simulink model "High_level_control_system"  (R2022b)
settings: Solver=VariableStepAuto  StartTime=0.0  StopTime=10.0  RelTol=1e-3
settings Model: Creator=louis  LastModifiedBy=simon
settings DebuggingCC: UnconnectedInputMsg=warning  UnconnectedOutputMsg=warning  UnconnectedLineMsg=warning
settings ModelReferenceCC: EnableRefExpFcnMdlSchedulingChecks=on
settings RTWCC: DLArmComputeVersion=19.05

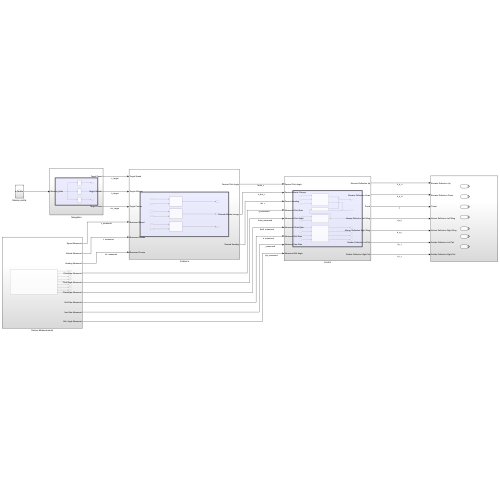
[thumbnail: Simulink's stored preview of the top-level diagram]
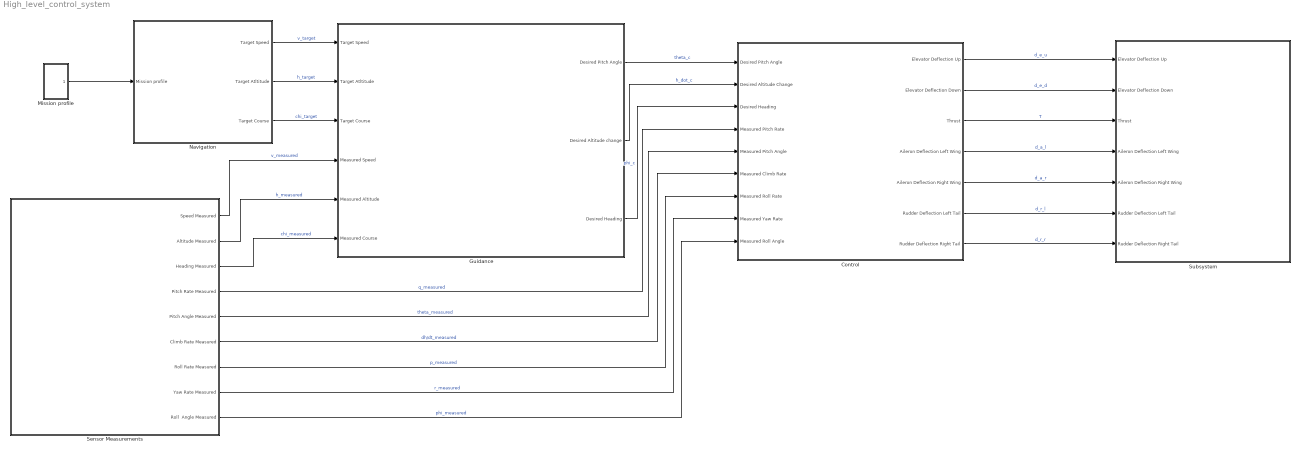
== system High_level_control_system ==
  Control : Subsystem
  Guidance : Subsystem
  Mission profile : Subsystem
  Navigation : Subsystem
  Sensor Measurements : Subsystem
  Subsystem : Subsystem
  wires:
  Navigation/1(Target Speed) -> Guidance/1(Target Speed)  "v_target"
  Navigation/2(Target Atltitude) -> Guidance/2(Target Atltitude)  "h_target"
  Navigation/3(Target Course) -> Guidance/3(Target Course)  "chi_target"
  Guidance/3(Desired Heading) -> Control/3(Desired Heading)  "phi_c"
  Guidance/2(Desired Altitude change) -> Control/2(Desired Altitude Change)  "h_dot_c"
  Guidance/1(Desired Pitch Angle) -> Control/1(Desired Pitch Angle)  "theta_c"
  Control/1(Elevator Deflection Up) -> Subsystem/1(Elevator Deflection Up)  "d_e_u"
  Control/3(Thrust) -> Subsystem/3(Thrust)  "T"
  Control/2(Elevator Deflection Down) -> Subsystem/2(Elevator Deflection Down)  "d_e_d"
  Control/4(Aileron Deflection Left Wing) -> Subsystem/4(Aileron Deflection Left Wing)  "d_a_l"
  Control/6(Rudder Deflection Left Tail) -> Subsystem/6(Rudder Deflection Left Tail)  "d_r_l"
  Control/5(Aileron Deflection Right Wing) -> Subsystem/5(Aileron Deflection Right Wing)  "d_a_r"
  Control/7(Rudder Deflection Right Tail) -> Subsystem/7(Rudder Deflection Right Tail)  "d_r_r"
  Sensor Measurements/1(Speed Measured) -> Guidance/4(Measured Speed)  "v_measured"
  Sensor Measurements/5(Pitch Angle Measured) -> Control/5(Measured Pitch Angle)  "theta_measured"
  Sensor Measurements/4(Pitch Rate Measured) -> Control/4(Measured Pitch Rate)  "q_measured"
  Sensor Measurements/3(Heading Measured) -> Guidance/6(Measured Course)  "chi_measured"
  Sensor Measurements/7(Roll Rate Measured) -> Control/7(Measured Roll Rate)  "p_measured"
  Sensor Measurements/8(Yaw Rate Measured) -> Control/8(Measured Yaw Rate)  "r_measured"
  Sensor Measurements/2(Altitude Measured) -> Guidance/5(Measured Altitude)  "h_measured"
  Sensor Measurements/9(Roll  Angle Measured) -> Control/9(Measured Roll Angle)  "phi_measured"
  Sensor Measurements/6(Climb Rate Measured) -> Control/6(Measured Climb Rate)  "dh/dt_measured"
  Mission profile/1(Mission profile) -> Navigation/1(Mission profile)

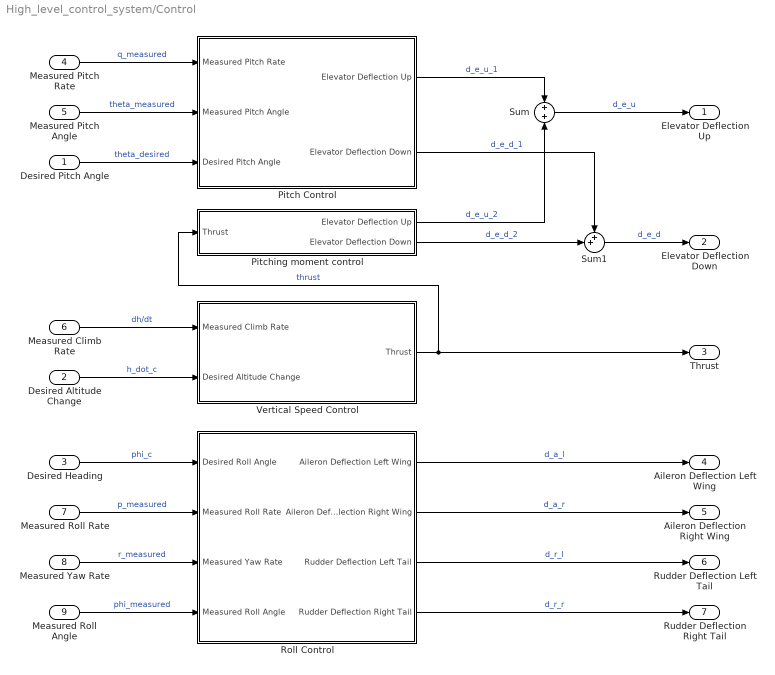
== system High_level_control_system/Control ==
  Desired Pitch Angle : Inport
  Desired Altitude Change : Inport  Port=2
  Desired Heading : Inport  Port=3
  Measured Pitch Rate : Inport  Port=4
  Measured Pitch Angle : Inport  Port=5
  Measured Climb Rate : Inport  Port=6
  Measured Roll Rate : Inport  Port=7
  Measured Yaw Rate : Inport  Port=8
  Measured Roll Angle : Inport  Port=9
  Pitch Control : Subsystem
  Pitching moment control : Subsystem
  Roll Control : Subsystem
  Sum : Sum
  Sum1 : Sum  Inputs=++|
  Vertical Speed Control : Subsystem
  Elevator Deflection Up : Outport
  Elevator Deflection Down : Outport  Port=2
  Thrust : Outport  Port=3
  Aileron Deflection Left Wing : Outport  Port=4
  Aileron Deflection Right Wing : Outport  Port=5
  Rudder Deflection Left Tail : Outport  Port=6
  Rudder Deflection Right Tail : Outport  Port=7
  wires:
  Pitch Control/1(Elevator Deflection Up) -> Sum/1  "d_e_u_1"
  Measured Pitch Rate/1 -> Pitch Control/1(Measured Pitch Rate)  "q_measured"
  Measured Pitch Angle/1 -> Pitch Control/2(Measured Pitch Angle)  "theta_measured"
  Desired Pitch Angle/1 -> Pitch Control/3(Desired Pitch Angle)  "theta_desired"
  Vertical Speed Control/1(Thrust) -> Pitching moment control/1(Thrust), Thrust/1  "thrust"
  Pitching moment control/1(Elevator Deflection Up) -> Sum/2  "d_e_u_2"
  Measured Climb Rate/1 -> Vertical Speed Control/1(Measured Climb Rate)  "dh/dt"
  Desired Altitude Change/1 -> Vertical Speed Control/2(Desired Altitude Change)  "h_dot_c"
  Desired Heading/1 -> Roll Control/1("Desired Roll Angle ")  "phi_c"
  Measured Roll Rate/1 -> Roll Control/2(Measured Roll Rate)  "p_measured"
  Measured Yaw Rate/1 -> Roll Control/3(Measured Yaw Rate)  "r_measured"
  Measured Roll Angle/1 -> Roll Control/4(Measured Roll Angle)  "phi_measured"
  Roll Control/3(Rudder Deflection Left Tail) -> Rudder Deflection Left Tail/1  "d_r_l"
  Roll Control/1(Aileron Deflection Left Wing) -> Aileron Deflection Left Wing/1  "d_a_l"
  Roll Control/2(Aileron Deflection Right Wing) -> Aileron Deflection Right Wing/1  "d_a_r"
  Roll Control/4(Rudder Deflection Right Tail) -> Rudder Deflection Right Tail/1  "d_r_r"
  Sum/1 -> Elevator Deflection Up/1  "d_e_u"
  Sum1/1 -> Elevator Deflection Down/1  "d_e_d"
  Pitching moment control/2(Elevator Deflection Down) -> Sum1/2  "d_e_d_2"
  Pitch Control/2(Elevator Deflection Down) -> Sum1/1  "d_e_d_1"

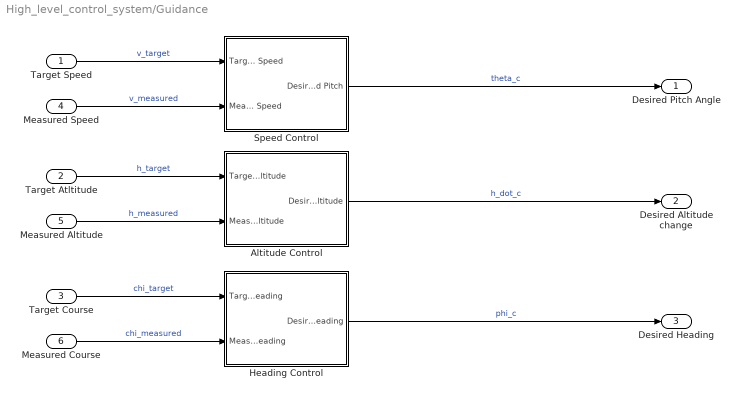
== system High_level_control_system/Guidance ==
  Target Speed : Inport
  Target Atltitude : Inport  Port=2
  Target Course : Inport  Port=3
  Measured Speed : Inport  Port=4
  Measured Altitude : Inport  Port=5
  Measured Course : Inport  Port=6
  Altitude Control : Subsystem
  Heading Control : Subsystem
  Speed Control : Subsystem
  Desired Pitch Angle : Outport
  Desired Altitude change : Outport  Port=2
  Desired Heading : Outport  Port=3
  wires:
  Target Speed/1 -> Speed Control/1(Target Speed)  "v_target"
  Measured Speed/1 -> Speed Control/2(Measured Speed)  "v_measured"
  Speed Control/1(Desired Pitch) -> Desired Pitch Angle/1  "theta_c"
  Target Atltitude/1 -> Altitude Control/1(Target Altitude)  "h_target"
  Measured Altitude/1 -> Altitude Control/2(Measured Altitude)  "h_measured"
  Altitude Control/1(Desired Altitude) -> Desired Altitude change/1  "h_dot_c"
  Heading Control/1(Desired Heading) -> Desired Heading/1  "phi_c"
  Measured Course/1 -> Heading Control/2(Measured Heading)  "chi_measured"
  Target Course/1 -> Heading Control/1(Target Heading)  "chi_target"

== system High_level_control_system/Mission profile ==
  Mission profile : Outport

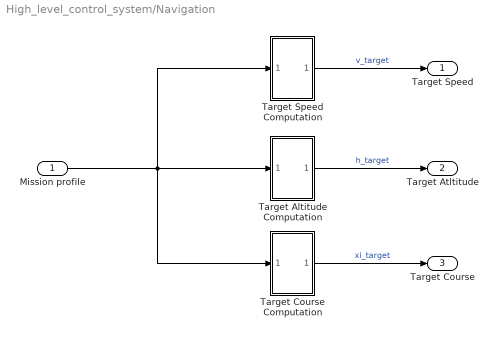
== system High_level_control_system/Navigation ==
  Mission profile : Inport
  Target Altitude Computation : Subsystem
  Target Course Computation : Subsystem
  Target Speed Computation : Subsystem
  Target Speed : Outport
  Target Atltitude : Outport  Port=2
  Target Course : Outport  Port=3
  wires:
  Mission profile/1 -> Target Speed Computation/1(In1), Target Altitude Computation/1(In1), Target Course Computation/1(In1)
  Target Speed Computation/1(Out1) -> Target Speed/1  "v_target"
  Target Altitude Computation/1(Out1) -> Target Atltitude/1  "h_target"
  Target Course Computation/1(Out1) -> Target Course/1  "xi_target"

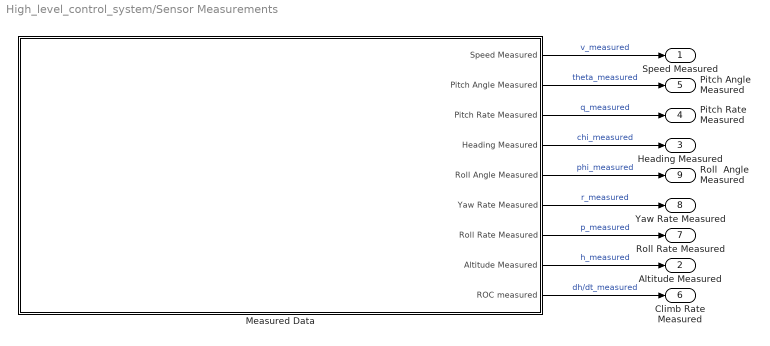
== system High_level_control_system/Sensor Measurements ==
  Measured Data : Subsystem
  Speed Measured : Outport
  Altitude Measured : Outport  Port=2
  Heading Measured : Outport  Port=3
  Pitch Rate Measured : Outport  Port=4
  Pitch Angle Measured : Outport  Port=5
  Climb Rate Measured : Outport  Port=6
  Roll Rate Measured : Outport  Port=7
  Yaw Rate Measured : Outport  Port=8
  Roll  Angle Measured : Outport  Port=9
  wires:
  Measured Data/7(Roll Rate Measured) -> Roll Rate Measured/1  "p_measured"
  Measured Data/6(Yaw Rate Measured) -> Yaw Rate Measured/1  "r_measured"
  Measured Data/5(Roll Angle Measured) -> Roll  Angle Measured/1  "phi_measured"
  Measured Data/2(Pitch Angle Measured) -> Pitch Angle Measured/1  "theta_measured"
  Measured Data/3(Pitch Rate Measured) -> Pitch Rate Measured/1  "q_measured"
  Measured Data/1(Speed Measured) -> Speed Measured/1  "v_measured"
  Measured Data/4(Heading Measured) -> Heading Measured/1  "chi_measured"
  Measured Data/8(Altitude Measured) -> Altitude Measured/1  "h_measured"
  Measured Data/9(ROC measured) -> Climb Rate Measured/1  "dh/dt_measured"

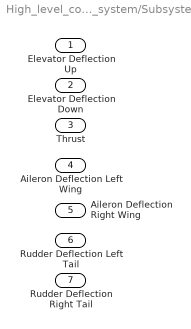
== system High_level_control_system/Subsystem ==
  Elevator Deflection Up : Inport
  Elevator Deflection Down : Inport  Port=2
  Thrust : Inport  Port=3
  Aileron Deflection Left Wing : Inport  Port=4
  Aileron Deflection Right Wing : Inport  Port=5
  Rudder Deflection Left Tail : Inport  Port=6
  Rudder Deflection Right Tail : Inport  Port=7

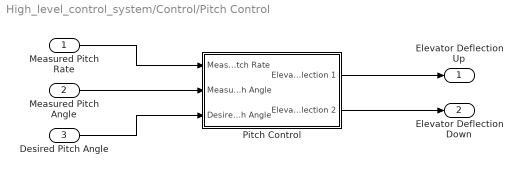
== system High_level_control_system/Control/Pitch Control ==
  Measured Pitch Rate : Inport
  Measured Pitch Angle : Inport  Port=2
  Desired Pitch Angle : Inport  Port=3
  Pitch Control : Subsystem
  Elevator Deflection Up : Outport
  Elevator Deflection Down : Outport  Port=2
  wires:
  Pitch Control/1(Elevator Deflection 1) -> Elevator Deflection Up/1
  Measured Pitch Rate/1 -> Pitch Control/1(Measured Pitch Rate)
  Measured Pitch Angle/1 -> Pitch Control/2(Measured Pitch Angle)
  Desired Pitch Angle/1 -> Pitch Control/3(Desired Pitch Angle)
  Pitch Control/2(Elevator Deflection 2) -> Elevator Deflection Down/1

== system High_level_control_system/Control/Pitching moment control ==
  Thrust : Inport
  Elevator Deflection Up : Outport
  Elevator Deflection Down : Outport  Port=2
  wires:
  Thrust/1 -> Elevator Deflection Up/1

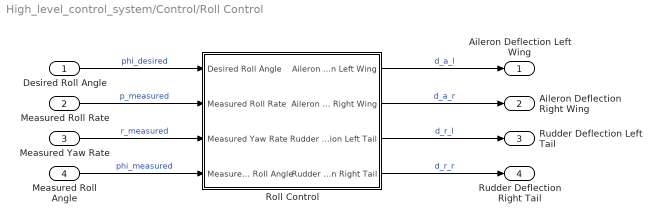
== system High_level_control_system/Control/Roll Control ==
  "Desired Roll Angle " : Inport
  Measured Roll Rate : Inport  Port=2
  Measured Yaw Rate : Inport  Port=3
  Measured Roll Angle : Inport  Port=4
  Roll Control : Subsystem
  Aileron Deflection Left Wing : Outport
  Aileron Deflection Right Wing : Outport  Port=2
  Rudder Deflection Left Tail : Outport  Port=3
  Rudder Deflection Right Tail : Outport  Port=4
  wires:
  Roll Control/1(Aileron Deflection Left Wing) -> Aileron Deflection Left Wing/1  "d_a_l"
  "Desired Roll Angle "/1 -> Roll Control/1(Desired Roll Angle)  "phi_desired"
  Measured Roll Rate/1 -> Roll Control/2(Measured Roll Rate)  "p_measured"
  Measured Yaw Rate/1 -> Roll Control/3(Measured Yaw Rate)  "r_measured"
  Measured Roll Angle/1 -> Roll Control/4(Measured Roll Angle)  "phi_measured"
  Roll Control/3(Rudder Deflection Left Tail) -> Rudder Deflection Left Tail/1  "d_r_l"
  Roll Control/2(Aileron Deflection Right Wing) -> Aileron Deflection Right Wing/1  "d_a_r"
  Roll Control/4(Rudder Deflection Right Tail) -> Rudder Deflection Right Tail/1  "d_r_r"

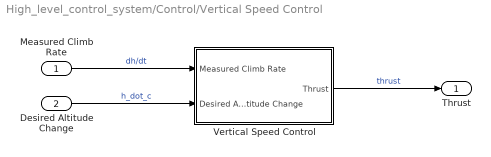
== system High_level_control_system/Control/Vertical Speed Control ==
  Measured Climb Rate : Inport
  Desired Altitude Change : Inport  Port=2
  Vertical Speed Control : Subsystem
  Thrust : Outport
  wires:
  Vertical Speed Control/1(Thrust) -> Thrust/1  "thrust"
  Measured Climb Rate/1 -> Vertical Speed Control/1(Measured Climb Rate)  "dh/dt"
  Desired Altitude Change/1 -> Vertical Speed Control/2(Desired Altitude Change)  "h_dot_c"

== system High_level_control_system/Guidance/Altitude Control ==
  Target Altitude : Inport
  Measured Altitude : Inport  Port=2
  Altitude Control : Subsystem
  Desired Altitude : Outport
  wires:
  Target Altitude/1 -> Altitude Control/1(Target Altitude)  "h_target"
  Measured Altitude/1 -> Altitude Control/2(Measured Altitude)  "h_measured"
  Altitude Control/1(Desired Altitude) -> Desired Altitude/1  "h_desired"

== system High_level_control_system/Guidance/Heading Control ==
  Target Heading : Inport
  Measured Heading : Inport  Port=2
  Heading Control : Subsystem
  Desired Heading : Outport
  wires:
  Target Heading/1 -> Heading Control/1(Target Heading)  "xi_target"
  Measured Heading/1 -> Heading Control/2(Measured Heading)  "xi_measured"
  Heading Control/1(Desired Heading) -> Desired Heading/1  "xi_desired"

== system High_level_control_system/Guidance/Speed Control ==
  Target Speed : Inport
  Measured Speed : Inport  Port=2
  Subsystem : Subsystem
  Desired Pitch : Outport
  wires:
  Target Speed/1 -> Subsystem/1(Target Speed)
  Measured Speed/1 -> Subsystem/2(Measured Speed)
  Subsystem/1(Desired Pitch) -> Desired Pitch/1

== system High_level_control_system/Navigation/Target Altitude Computation ==
  In1 : Inport
  Out1 : Outport
  wires:
  In1/1 -> Out1/1

== system High_level_control_system/Navigation/Target Course Computation ==
  In1 : Inport
  Out1 : Outport
  wires:
  In1/1 -> Out1/1

== system High_level_control_system/Navigation/Target Speed Computation ==
  In1 : Inport
  Out1 : Outport
  wires:
  In1/1 -> Out1/1

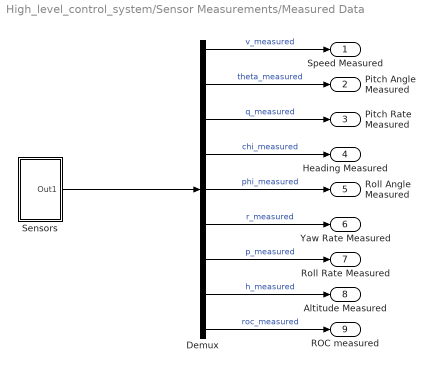
== system High_level_control_system/Sensor Measurements/Measured Data ==
  Demux : Demux  Outputs=9
  Sensors : Subsystem
  Speed Measured : Outport
  Pitch Angle Measured : Outport  Port=2
  Pitch Rate Measured : Outport  Port=3
  Heading Measured : Outport  Port=4
  Roll Angle Measured : Outport  Port=5
  Yaw Rate Measured : Outport  Port=6
  Roll Rate Measured : Outport  Port=7
  Altitude Measured : Outport  Port=8
  ROC measured : Outport  Port=9
  wires:
  Demux/7 -> Roll Rate Measured/1  "p_measured"
  Demux/3 -> Pitch Rate Measured/1  "q_measured"
  Demux/5 -> Roll Angle Measured/1  "phi_measured"
  Demux/6 -> Yaw Rate Measured/1  "r_measured"
  Demux/1 -> Speed Measured/1  "v_measured"
  Demux/4 -> Heading Measured/1  "chi_measured"
  Demux/2 -> Pitch Angle Measured/1  "theta_measured"
  Sensors/1(Out1) -> Demux/1
  Demux/8 -> Altitude Measured/1  "h_measured"
  Demux/9 -> ROC measured/1  "roc_measured"

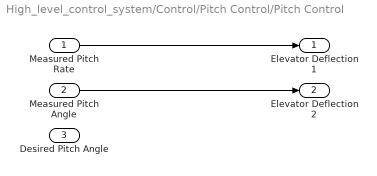
== system High_level_control_system/Control/Pitch Control/Pitch Control ==
  Measured Pitch Rate : Inport
  Measured Pitch Angle : Inport  Port=2
  Desired Pitch Angle : Inport  Port=3
  Elevator Deflection 1 : Outport
  Elevator Deflection 2 : Outport  Port=2
  wires:
  Measured Pitch Rate/1 -> Elevator Deflection 1/1
  Measured Pitch Angle/1 -> Elevator Deflection 2/1

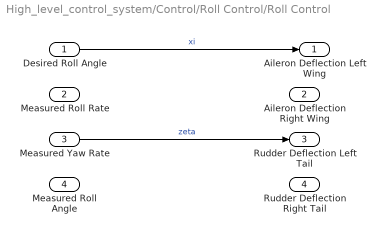
== system High_level_control_system/Control/Roll Control/Roll Control ==
  Desired Roll Angle : Inport
  Measured Roll Rate : Inport  Port=2
  Measured Yaw Rate : Inport  Port=3
  Measured Roll Angle : Inport  Port=4
  Aileron Deflection Left Wing : Outport
  Aileron Deflection Right Wing : Outport  Port=2
  Rudder Deflection Left Tail : Outport  Port=3
  Rudder Deflection Right Tail : Outport  Port=4
  wires:
  Desired Roll Angle/1 -> Aileron Deflection Left Wing/1  "xi"
  Measured Yaw Rate/1 -> Rudder Deflection Left Tail/1  "zeta"

== system High_level_control_system/Control/Vertical Speed Control/Vertical Speed Control ==
  Measured Climb Rate : Inport
  Desired Altitude Change : Inport  Port=2
  Thrust : Outport
  wires:
  Measured Climb Rate/1 -> Thrust/1

== system High_level_control_system/Guidance/Altitude Control/Altitude Control ==
  Target Altitude : Inport
  Measured Altitude : Inport  Port=2
  Desired Altitude : Outport
  wires:
  Target Altitude/1 -> Desired Altitude/1

== system High_level_control_system/Guidance/Heading Control/Heading Control ==
  Target Heading : Inport
  Measured Heading : Inport  Port=2
  Desired Heading : Outport
  wires:
  Target Heading/1 -> Desired Heading/1

== system High_level_control_system/Guidance/Speed Control/Subsystem ==
  Target Speed : Inport
  Measured Speed : Inport  Port=2
  Desired Pitch : Outport
  wires:
  Target Speed/1 -> Desired Pitch/1

== system High_level_control_system/Sensor Measurements/Measured Data/Sensors ==
  note: Sensors
  Out1 : Outport
